simulink model "simulacao_com_observador"  (R2020a)
settings: Solver=ode45  StartTime=0.0  StopTime=15.0  RelTol=1e-3  EnableMultiTasking=on
values from neighbouring files (symbols this model uses):
  C = [1 0]    [trabalho_final.m]
  delta = mb*L*L + Ib    (= 0.00848237644)    [trabalho_final.m]
  g = 9.81    [trabalho_final.m]
  gamah = mb*L    (= 0.039903)    [trabalho_final.m]
  K = place(phi, gama, polos)    [trabalho_final.m]
  Kec = inv(phi)*Kep    [trabalho_final.m]
  Ta = 2*pi/ws    [trabalho_final.m]
undefined symbols (not defined in the file or in its folder): gama, phi
settings Model: Creator=arthu  LastModifiedBy=Acer
settings DataIOCC: LimitDataPoints=on  SaveFormat=Array  ReturnWorkspaceOutputs=off
settings OptimizationCC: LifeSpan=inf
settings DebuggingCC: SFUnexpectedBacktrackingDiag=warning  SFNoUnconditionalDefaultTransitionDiag=warning  SFExecutionAtInitializationDiag=none  ArithmeticOperatorsInVariantConditions=warning
settings HardwareCC: ProdBitPerPointer=32  ProdBitPerSizeT=32  ProdBitPerPtrDiffT=32  ProdLargestAtomicFloat=None  ProdIntDivRoundTo=Undefined  ProdEndianess=Unspecified  ProdWordSize=32  ProdHWDeviceType=32-bit Generic
settings ModelReferenceCC: PropagateSignalLabelsOutOfModel=off
settings SFSimCC: SimUseLocalCustomCode=off  CustomCodeUndefinedFunction=UseInterfaceOnly
settings RTWCC: RTWUseLocalCustomCode=off
settings CodeAppCC: StateflowObjectComments=on
settings GRTTargetCC: TargetLangStandard=C89/C90 (ANSI)
settings ConfigComp: CovMetricSettings=dw  CovHtmlReporting=on  CovSaveCumulativeToWorkspaceVar=on  CovSaveSingleToWorkspaceVar=on  CovExternalEMLEnable=off

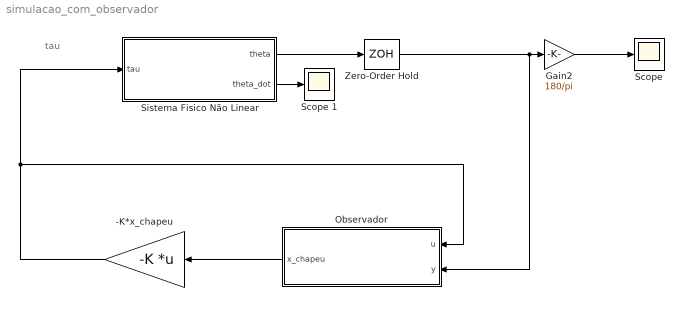
== system simulacao_com_observador ==
  note: tau
  -K*x_chapeu : Gain  Gain=-K  Multiplication=Matrix(K*u)
  Gain2 : Gain  Gain=180/pi
  Observador : Subsystem
  "Scope " : Scope
  Scope 1 : Scope
  Sistema Fisico Não Linear : Subsystem
  Zero-Order Hold : ZeroOrderHold  SampleTime=Ta
  wires:
  Sistema Fisico Não Linear/1(theta) -> Zero-Order Hold/1
  Zero-Order Hold/1 -> Observador/2(y), Gain2/1
  -K*x_chapeu/1 -> Observador/1(u), Sistema Fisico Não Linear/1(tau)
  Gain2/1 -> "Scope "/1
  Observador/1(x_chapeu) -> -K*x_chapeu/1
  Sistema Fisico Não Linear/2(theta_dot) -> Scope 1/1

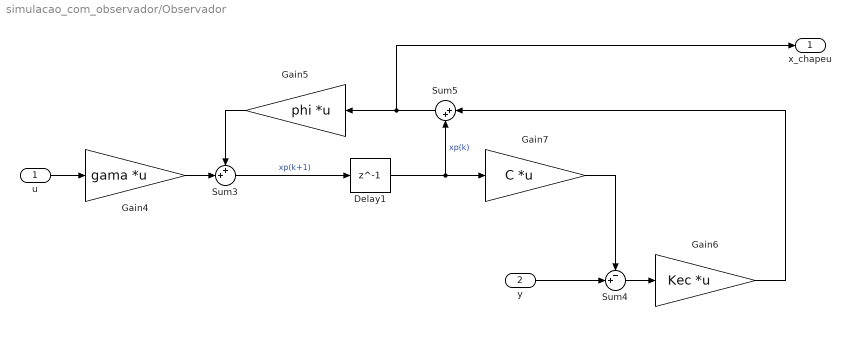
== system simulacao_com_observador/Observador ==
  u : Inport
  y : Inport  Port=2
  Delay1 : Delay  DelayLength=1  InitialCondition=[0;0]
  Gain4 : Gain  Gain=gama  Multiplication=Matrix(K*u) (u vector)
  Gain5 : Gain  Gain=phi  Multiplication=Matrix(K*u) (u vector)
  Gain6 : Gain  Gain=Kec  Multiplication=Matrix(K*u) (u vector)
  Gain7 : Gain  Gain=C  Multiplication=Matrix(K*u) (u vector)
  Sum3 : Sum  Inputs=++|
  Sum4 : Sum  Inputs=-+|
  Sum5 : Sum  Inputs=|++
  x_chapeu : Outport  VectorParamsAs1DForOutWhenUnconnected=off
  wires:
  Gain6/1 -> Sum5/1
  Sum3/1 -> Delay1/1  "xp(k+1)"
  u/1 -> Gain4/1
  Gain4/1 -> Sum3/2
  Delay1/1 -> Gain7/1, Sum5/2  "xp(k)"
  Gain5/1 -> Sum3/1
  Sum4/1 -> Gain6/1
  Gain7/1 -> Sum4/1
  y/1 -> Sum4/2
  Sum5/1 -> x_chapeu/1, Gain5/1

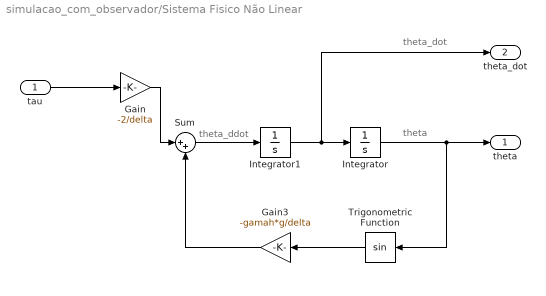
== system simulacao_com_observador/Sistema Fisico Não Linear ==
  note: theta
  note: theta_dot
  note: theta_ddot
  tau : Inport
  Gain : Gain  Gain=-2/delta
  Gain3 : Gain  Gain=-gamah*g/delta
  Integrator : Integrator  InitialCondition=20*pi/180
  Integrator1 : Integrator
  Sum : Sum  Inputs=|++
  Trigonometric Function : Trigonometry
  theta : Outport
  theta_dot : Outport  Port=2
  wires:
  tau/1 -> Gain/1
  Sum/1 -> Integrator1/1
  Gain3/1 -> Sum/2
  Integrator/1 -> theta/1, Trigonometric Function/1
  Trigonometric Function/1 -> Gain3/1
  Gain/1 -> Sum/1
  Integrator1/1 -> theta_dot/1, Integrator/1
